simulink model "Simulink_Model"  (R2018a)
settings: Solver=VariableStepAuto  StartTime=0.0  StopTime=T_v(n+1)  MaxStep=0.001
values from neighbouring files (symbols this model uses):
  euler_v = deg2rad(euler_v)    [Simulation_Parameters.m]
  I_b = [151612935.5/10^9	       -12035.62/10^9        -9941.66/10^9 ... (first row only)    [Simulation_Parameters.m]
  I_new = I_sys - I_rw_z * (a1_R1_to_0*a1_0_to_R1+a2_R2_to_0*a2_0_to_R2+a3_R3_to_0*a3_0_to_R3)    [Simulation_Parameters.m]
  I_rw_z = 418129.72/10^9    (= 0.00041812972)    [Simulation_Parameters.m]
  I_single_rw = [220358.07/10^9         0               0 ... (first row only)    [Simulation_Parameters.m]
  I_st = [118601552.74/10^9	       -491524.85/10^9         95420.21/10^9 ... (first row only)    [Simulation_Parameters.m]
  I_sys = [177776253.6/10^9         -12078.47/10^9	        -9914.94/10^9 ... (first row only)    [Simulation_Parameters.m]
  Kd_r = [d;d;d]    [Simulation_Parameters.m]
  Kd_t = [d;d]    [Simulation_Parameters.m]
  Kp_r = [p;p;p]    [Simulation_Parameters.m]
  Kp_t = [p;p]    [Simulation_Parameters.m]
  m_b = 16.9927    [Simulation_Parameters.m]
  m_rw = 0.24806    [Simulation_Parameters.m]
  m_st = 9.48989    [Simulation_Parameters.m]
  m_tot = m_sys + m_st    (= 27.22678)    [Simulation_Parameters.m]
  mf = 1    [Simulation_Parameters.m]
  n = 4    [Simulation_Parameters.m]
  R_0_to_1 = [sqrt(2)/2 0.5 0.5; -sqrt(2)/2 0.5 0.5; 0 -sqrt(2)/2 sqrt(2)/2]    [Simulation_Parameters.m]
  R_1_to_0 = inv(R_0_to_1)    [Simulation_Parameters.m]
undefined symbols (not defined in the file or in its folder): k_phi_1, k_phi_2, k_phi_3, k_psi_1, k_psi_2, k_psi_3, k_theta_1, k_theta_2, k_theta_3, k_x_1, k_x_2, k_x_3, k_y_1, k_y_2, k_y_3, pos_v, t_acc, t_no_acc, t_t_acc, t_t_no_acc, T_v, X, Y, Z
libraries: nesl_utility x20, sm_lib x16, vrlib x2
(part 1 of 2)
settings Model: Creator=menel  LastModifiedBy=Menelaos
settings SolverCC: MaxConsecutiveZCs=10000  ShapePreserveControl=EnableAll  ZeroCrossAlgorithm=Adaptive  AlgebraicLoopSolver=LineSearch
settings DebuggingCC: MaxConsecutiveZCsMsg=none

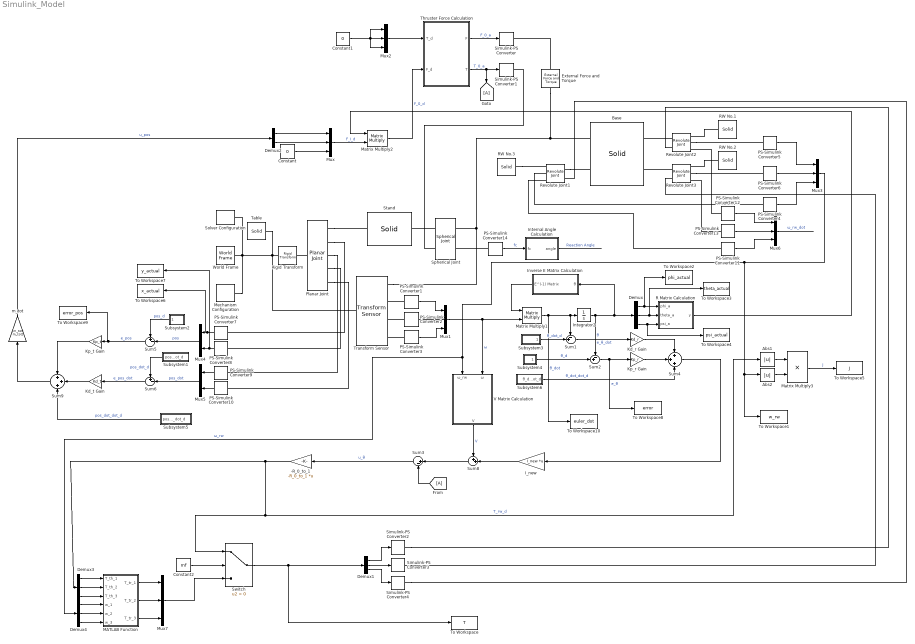
== system Simulink_Model ==
  -R_0_to_1 : Gain  Gain=-R_0_to_1  Multiplication=Matrix(K*u) (u vector)
  Abs1 : Abs
  Abs2 : Abs
  Base : sm_lib/Body Elements/Solid  InertiaType=Custom  Mass=m_b  MassUnits=kg  CenterOfMass=COM_b  CenterOfMassUnits=m  MomentsOfInertia=[I_b(1,1) I_b(2,2) I_b(3,3)]  MomentsOfInertiaUnits=kg*m^2  ProductsOfInertia=[I_b(2,3) I_b(1,3) I_b(2,1)]  ProductsOfInertiaUnits=kg*m^2  DensityBased=off  Density=1000  DensityUnits=kg/m^3  DoExposeReferenceFrame=on  SerializedFrames=<Frames><Frame><Id>Frame1</Id><Value><Name>wheel 1</Name><Origin><Source>GeometricFeature</Source><FeatureName>planar surface 30</FeatureName></Origin><PrimaryAxis><DefinedDirection>+Z</DefinedDirection><Source>GeometricFeature</Source><SourceDirection>+Z</SourceDirection><FeatureName>planar surface 30</FeatureName></PrimaryAxis><SecondaryAxis><DefinedDirection>+X</DefinedDirection><Source>ReferenceFrame</Source><SourceDirection>+X</SourceDirection><FeatureName></FeatureName></SecondaryAxis></Value></Frame><Frame><Id>Frame2</Id><Value><Name>wheel 2</Name><Origin><Source>GeometricFeature</Source><FeatureName>planar surface 29</FeatureName></Origin><PrimaryAxis><DefinedDirection>+Z</DefinedDirection><Source>GeometricFeature</Source><SourceDirection>+Z</SourceDirection><FeatureName>planar surface 29</FeatureName></PrimaryAxis><SecondaryAxis><DefinedDirection>+X</DefinedDirection><Source>ReferenceFrame</Source><SourceDirection>+X</SourceDirection><FeatureName></FeatureName></SecondaryAxis></Value></Frame><Frame><Id>Frame3</Id><Value><Name>wheel 3</Name><Origin><Source>GeometricFeature</Source><FeatureName>planar surface 31</FeatureName></Origin><PrimaryAxis><DefinedDirection>+Z</DefinedDirection><Source>GeometricFeature</Source><SourceDirection>+Z</SourceDirection><FeatureName>planar surface 31</FeatureName></PrimaryAxis><SecondaryAxis><DefinedDirection>+X</DefinedDirection><Source>ReferenceFrame</Source><SourceDirection>+X</SourceDirection><FeatureName></FeatureName></SecondaryAxis></Value></Frame></Frames>  GraphicType=FromGeometry  MarkerShape=Sphere  MarkerSize=10  GraphicVisPropType=SimpleVisualProperties  GraphicDiffuseColor=[0.6 0.6 1.0]  GraphicSpecularColor=[0.5 0.5 0.5 1.0]  GraphicAmbientColor=[0.15 0.15 0.15 1.0]  GraphicEmissiveColor=[0.0 0.0 0.0 1.0]  GraphicShininess=75  GraphicOpacity=1.0  GeometryShape=FromFile  RectangleSize=[1 1]  RectangleSizeUnits=m  BrickDimensions=[1 1 1]  BrickDimensionUnits=m  CylinderRadius=1  CylinderRadiusUnits=m  CylinderLength=1  CylinderLengthUnits=m  SphereRadius=1  SphereRadiusUnits=m  EllipsoidRadii=[1 1 1]  EllipsoidRadiiUnits=m  ExtrusionCrossSection=[1 1; -1 1; -1 -1; 1 -1]  ExtrusionCrossSectionUnits=m  ExtrusionLength=1  ExtrusionLengthUnits=m  PolygonNumSides=3  PolygonOuterRadius=1  PolygonOuterRadiusUnits=m  ExtGeomFileType=STEP  ExtGeomFileName=D:\School\Διπλωματική\Final_Delivery\Motion_and_Rotation_Simulation\Base.STEP  ExtGeomFileUnits=m  RevolutionCrossSection=[1 1; 1 -1; 2 -1; 2 1]  RevolutionCrossSectionUnits=m  RevolutionExtent=Full  RevolutionAngle=180  RevolutionAngleUnits=deg
  Constant : Constant  Value=0
  Constant1 : Constant  Value=0
  Constant2 : Constant  Value=mf
  Demux{,1,3..4} (4 alike) : Demux  Outputs=3
  Demux2 : Demux  Outputs=2
  External Force and Torque : sm_lib/Forces and Torques/External Force and Torque  ForceResolutionFrame=AttachedFrame  EnableForceX=off  EnableForceY=off  EnableForceZ=off  EnableForce=on  TorqueResolutionFrame=AttachedFrame  EnableTorqueX=off  EnableTorqueY=off  EnableTorqueZ=off  EnableTorque=off
  I_new : Gain  Gain=I_new  Multiplication=Matrix(K*u) (u vector)
  Integrator2 : Integrator
  Internal Angle Calculation : MATLAB Function  TreatAsAtomicUnit=on
  Inverse E Matrix Calculation : Subsystem
  Kd_r Gain : Gain  Gain=Kd_r
  Kd_t Gain : Gain  Gain=Kd_t
  Kp_r Gain : Gain  Gain=Kp_r
  Kp_t Gain : Gain  Gain=Kp_t
  MATLAB Function : MATLAB Function  TreatAsAtomicUnit=on
  Matrix Multiply1 : Product  Multiplication=Matrix(*)
  Matrix Multiply2 : Product  Multiplication=Matrix(*)
  Matrix Multiply3 : Product
  Mechanism Configuration : sm_lib/Utilities/Mechanism Configuration  UniformGravity=Constant  GravityVector=[0 0 0]  GravityUnits=m/s^2  LinearizationDelta=0.001
  Mux{,1..3,6..7} (6 alike) : Mux  Inputs=3
  Mux4 : Mux  Inputs=2
  Mux5 : Mux  Inputs=2
  PS-Simulink Converter{1..3,7..13} (10 alike) : nesl_utility/PS-Simulink Converter  PhysicalDomain=network_engine_domain  SubClassName=ps_output  LeftPortType=input  RightPortType=output  PseudoPeriodic=off  Frequencies=[]  Unit=1  AffineConversion=off
  PS-Simulink Converter14 : nesl_utility/PS-Simulink Converter  PhysicalDomain=network_engine_domain  SubClassName=ps_output  LeftPortType=input  RightPortType=output  PseudoPeriodic=off  Frequencies=[]  Unit=N  AffineConversion=off
  PS-Simulink Converter4 : nesl_utility/PS-Simulink Converter  PhysicalDomain=network_engine_domain  SubClassName=ps_output  LeftPortType=input  RightPortType=output  PseudoPeriodic=off  Frequencies=[]  Unit=rad/s  AffineConversion=off
  PS-Simulink Converter5 : nesl_utility/PS-Simulink Converter  PhysicalDomain=network_engine_domain  SubClassName=ps_output  LeftPortType=input  RightPortType=output  PseudoPeriodic=off  Frequencies=[]  Unit=rad/s  AffineConversion=off
  PS-Simulink Converter6 : nesl_utility/PS-Simulink Converter  PhysicalDomain=network_engine_domain  SubClassName=ps_output  LeftPortType=input  RightPortType=output  PseudoPeriodic=off  Frequencies=[]  Unit=rad/s  AffineConversion=off
  Planar Joint : sm_lib/Joints/Planar Joint  SenseConstraintForce=off  SenseConstraintForceX=off  SenseConstraintForceY=off  SenseConstraintForceZ=off  SenseConstraintTorque=off  SenseConstraintTorqueX=off  SenseConstraintTorqueY=off  SenseConstraintTorqueZ=off  SenseTotalForce=off  SenseTotalForceX=off  SenseTotalForceY=off  SenseTotalForceZ=off  SenseTotalTorque=off  SenseTotalTorqueX=off  SenseTotalTorqueY=off  SenseTotalTorqueZ=off  CompositeWrenchDir=FollowerOnBase  CompositeWrenchFrame=BaseFrame  PxEquilibriumPosition=0  PxEquilibriumPositionUnits=m  PxSpringStiffness=0  PxSpringStiffnessUnits=N/m  PxDampingCoefficient=0  PxDampingCoefficientUnits=N/(m/s)  PxTorqueActuationMode=NoTorque  PxMotionActuationMode=ComputedMotion  PxSensePosition=on  PxSenseVelocity=on  PxSenseAcceleration=off  PxSenseTorqueForce=off  PxPositionTargetSpecify=off  PxPositionTargetPriority=High  PxPositionTargetValue=0  PxPositionTargetValueUnits=m  PxVelocityTargetSpecify=off  PxVelocityTargetPriority=High  PxVelocityTargetValue=0  PxVelocityTargetValueUnits=m/s  PyEquilibriumPosition=0  PyEquilibriumPositionUnits=m  PySpringStiffness=0  PySpringStiffnessUnits=N/m  PyDampingCoefficient=0  PyDampingCoefficientUnits=N/(m/s)  PyTorqueActuationMode=NoTorque  PyMotionActuationMode=ComputedMotion  PySensePosition=on  PySenseVelocity=on  PySenseAcceleration=off  PySenseTorqueForce=off  PyPositionTargetSpecify=off  PyPositionTargetPriority=High  PyPositionTargetValue=0  PyPositionTargetValueUnits=m  PyVelocityTargetSpecify=off  PyVelocityTargetPriority=High  PyVelocityTargetValue=0  PyVelocityTargetValueUnits=m/s  RzEquilibriumPosition=0  RzEquilibriumPositionUnits=deg  RzSpringStiffness=100  RzSpringStiffnessUnits=N*m/deg  RzDampingCoefficient=100  RzDampingCoefficientUnits=N*m/(deg/s)  RzTorqueActuationMode=NoTorque  RzMotionActuationMode=ComputedMotion  RzSensePosition=off  RzSenseVelocity=off  RzSenseAcceleration=off  RzSenseTorqueForce=off  RzPositionTargetSpecify=off  RzPositionTargetPriority=High  RzPositionTargetValue=0  RzPositionTargetValueUnits=deg  RzVelocityTargetSpecify=off  RzVelocityTargetPriority=High  RzVelocityTargetValue=0  RzVelocityTargetValueUnits=deg/s
  R Matrix Calculation : MATLAB Function  TreatAsAtomicUnit=on
  RW No.1 : sm_lib/Body Elements/Solid  InertiaType=Custom  Mass=m_rw  MassUnits=kg  CenterOfMass=COM_rw  CenterOfMassUnits=m  MomentsOfInertia=[I_single_rw(1,1) I_single_rw(2,2) I_single_rw(3,3)]  MomentsOfInertiaUnits=kg*m^2  ProductsOfInertia=[I_single_rw(2,3) I_single_rw(1,3) I_single_rw(2,1)]  ProductsOfInertiaUnits=kg*m^2  DensityBased=off  Density=1000  DensityUnits=kg/m^3  DoExposeReferenceFrame=off  SerializedFrames=<Frames><Frame><Id>Frame1</Id><Value><Name>R</Name><Origin><Source>GeometricFeature</Source><FeatureName>planar surface 2</FeatureName></Origin><PrimaryAxis><DefinedDirection>+Z</DefinedDirection><Source>ReferenceFrame</Source><SourceDirection>+Z</SourceDirection><FeatureName></FeatureName></PrimaryAxis><SecondaryAxis><DefinedDirection>+X</DefinedDirection><Source>ReferenceFrame</Source><SourceDirection>+X</SourceDirection><FeatureName></FeatureName></SecondaryAxis></Value></Frame></Frames>  GraphicType=FromGeometry  MarkerShape=Sphere  MarkerSize=10  GraphicVisPropType=SimpleVisualProperties  GraphicDiffuseColor=[1.0 0.2 0.2]  GraphicSpecularColor=[0.5 0.5 0.5 1.0]  GraphicAmbientColor=[0.15 0.15 0.15 1.0]  GraphicEmissiveColor=[0.0 0.0 0.0 1.0]  GraphicShininess=75  GraphicOpacity=1.0  GeometryShape=FromFile  RectangleSize=[1 1]  RectangleSizeUnits=m  BrickDimensions=[1 1 1]  BrickDimensionUnits=m  CylinderRadius=1  CylinderRadiusUnits=m  CylinderLength=1  CylinderLengthUnits=m  SphereRadius=1  SphereRadiusUnits=m  EllipsoidRadii=[1 1 1]  EllipsoidRadiiUnits=m  ExtrusionCrossSection=[1 1; -1 1; -1 -1; 1 -1]  ExtrusionCrossSectionUnits=m  ExtrusionLength=1  ExtrusionLengthUnits=m  PolygonNumSides=3  PolygonOuterRadius=1  PolygonOuterRadiusUnits=m  ExtGeomFileType=STEP  ExtGeomFileName=D:\School\Διπλωματική\Final_Delivery\Motion_and_Rotation_Simulation\Reaction_Wheel.STEP  ExtGeomFileUnits=m  RevolutionCrossSection=[1 1; 1 -1; 2 -1; 2 1]  RevolutionCrossSectionUnits=m  RevolutionExtent=Full  RevolutionAngle=180  RevolutionAngleUnits=deg
  RW No.2 : sm_lib/Body Elements/Solid  InertiaType=Custom  Mass=m_rw  MassUnits=kg  CenterOfMass=COM_rw  CenterOfMassUnits=m  MomentsOfInertia=[I_single_rw(1,1) I_single_rw(2,2) I_single_rw(3,3)]  MomentsOfInertiaUnits=kg*m^2  ProductsOfInertia=[I_single_rw(2,3) I_single_rw(1,3) I_single_rw(2,1)]  ProductsOfInertiaUnits=kg*m^2  DensityBased=off  Density=1000  DensityUnits=kg/m^3  DoExposeReferenceFrame=off  SerializedFrames=<Frames><Frame><Id>Frame1</Id><Value><Name>R</Name><Origin><Source>GeometricFeature</Source><FeatureName>planar surface 2</FeatureName></Origin><PrimaryAxis><DefinedDirection>+Z</DefinedDirection><Source>ReferenceFrame</Source><SourceDirection>+Z</SourceDirection><FeatureName></FeatureName></PrimaryAxis><SecondaryAxis><DefinedDirection>+X</DefinedDirection><Source>ReferenceFrame</Source><SourceDirection>+X</SourceDirection><FeatureName></FeatureName></SecondaryAxis></Value></Frame></Frames>  GraphicType=FromGeometry  MarkerShape=Sphere  MarkerSize=10  GraphicVisPropType=SimpleVisualProperties  GraphicDiffuseColor=[1.0 0.2 0.2]  GraphicSpecularColor=[0.5 0.5 0.5 1.0]  GraphicAmbientColor=[0.15 0.15 0.15 1.0]  GraphicEmissiveColor=[0.0 0.0 0.0 1.0]  GraphicShininess=75  GraphicOpacity=1.0  GeometryShape=FromFile  RectangleSize=[1 1]  RectangleSizeUnits=m  BrickDimensions=[1 1 1]  BrickDimensionUnits=m  CylinderRadius=1  CylinderRadiusUnits=m  CylinderLength=1  CylinderLengthUnits=m  SphereRadius=1  SphereRadiusUnits=m  EllipsoidRadii=[1 1 1]  EllipsoidRadiiUnits=m  ExtrusionCrossSection=[1 1; -1 1; -1 -1; 1 -1]  ExtrusionCrossSectionUnits=m  ExtrusionLength=1  ExtrusionLengthUnits=m  PolygonNumSides=3  PolygonOuterRadius=1  PolygonOuterRadiusUnits=m  ExtGeomFileType=STEP  ExtGeomFileName=D:\School\Διπλωματική\Final_Delivery\Motion_and_Rotation_Simulation\Reaction_Wheel.STEP  ExtGeomFileUnits=m  RevolutionCrossSection=[1 1; 1 -1; 2 -1; 2 1]  RevolutionCrossSectionUnits=m  RevolutionExtent=Full  RevolutionAngle=180  RevolutionAngleUnits=deg
  RW No.3 : sm_lib/Body Elements/Solid  InertiaType=Custom  Mass=m_rw  MassUnits=kg  CenterOfMass=COM_rw  CenterOfMassUnits=m  MomentsOfInertia=[I_single_rw(1,1) I_single_rw(2,2) I_single_rw(3,3)]  MomentsOfInertiaUnits=kg*m^2  ProductsOfInertia=[I_single_rw(2,3) I_single_rw(1,3) I_single_rw(2,1)]  ProductsOfInertiaUnits=kg*m^2  DensityBased=off  Density=1000  DensityUnits=kg/m^3  DoExposeReferenceFrame=off  SerializedFrames=<Frames><Frame><Id>Frame1</Id><Value><Name>R</Name><Origin><Source>GeometricFeature</Source><FeatureName>planar surface 2</FeatureName></Origin><PrimaryAxis><DefinedDirection>+Z</DefinedDirection><Source>ReferenceFrame</Source><SourceDirection>+Z</SourceDirection><FeatureName></FeatureName></PrimaryAxis><SecondaryAxis><DefinedDirection>+X</DefinedDirection><Source>ReferenceFrame</Source><SourceDirection>+X</SourceDirection><FeatureName></FeatureName></SecondaryAxis></Value></Frame></Frames>  GraphicType=FromGeometry  MarkerShape=Sphere  MarkerSize=10  GraphicVisPropType=SimpleVisualProperties  GraphicDiffuseColor=[1.0 0.2 0.2]  GraphicSpecularColor=[0.5 0.5 0.5 1.0]  GraphicAmbientColor=[0.15 0.15 0.15 1.0]  GraphicEmissiveColor=[0.0 0.0 0.0 1.0]  GraphicShininess=75  GraphicOpacity=1.0  GeometryShape=FromFile  RectangleSize=[1 1]  RectangleSizeUnits=m  BrickDimensions=[1 1 1]  BrickDimensionUnits=m  CylinderRadius=1  CylinderRadiusUnits=m  CylinderLength=1  CylinderLengthUnits=m  SphereRadius=1  SphereRadiusUnits=m  EllipsoidRadii=[1 1 1]  EllipsoidRadiiUnits=m  ExtrusionCrossSection=[1 1; -1 1; -1 -1; 1 -1]  ExtrusionCrossSectionUnits=m  ExtrusionLength=1  ExtrusionLengthUnits=m  PolygonNumSides=3  PolygonOuterRadius=1  PolygonOuterRadiusUnits=m  ExtGeomFileType=STEP  ExtGeomFileName=D:\School\Διπλωματική\Final_Delivery\Motion_and_Rotation_Simulation\Reaction_Wheel.STEP  ExtGeomFileUnits=m  RevolutionCrossSection=[1 1; 1 -1; 2 -1; 2 1]  RevolutionCrossSectionUnits=m  RevolutionExtent=Full  RevolutionAngle=180  RevolutionAngleUnits=deg
  Revolute Joint1 : sm_lib/Joints/Revolute Joint  SenseConstraintForce=off  SenseConstraintForceX=off  SenseConstraintForceY=off  SenseConstraintForceZ=off  SenseConstraintTorque=off  SenseConstraintTorqueX=off  SenseConstraintTorqueY=off  SenseConstraintTorqueZ=off  SenseTotalForce=off  SenseTotalForceX=off  SenseTotalForceY=off  SenseTotalForceZ=off  SenseTotalTorque=off  SenseTotalTorqueX=off  SenseTotalTorqueY=off  SenseTotalTorqueZ=off  CompositeWrenchDir=FollowerOnBase  CompositeWrenchFrame=BaseFrame  EquilibriumPosition=0  EquilibriumPositionUnits=deg  SpringStiffness=0  SpringStiffnessUnits=N*m/deg  DampingCoefficient=1.86*10^(-5)  DampingCoefficientUnits=N*m/(rad/s)  TorqueActuationMode=InputTorque  MotionActuationMode=ComputedMotion  SensePosition=off  SenseVelocity=on  SenseAcceleration=on  SenseTorqueForce=off  PositionTargetSpecify=on  PositionTargetPriority=High  PositionTargetValue=0  PositionTargetValueUnits=deg  VelocityTargetSpecify=off  VelocityTargetPriority=High  VelocityTargetValue=300  VelocityTargetValueUnits=rad/s
  Revolute Joint2 : sm_lib/Joints/Revolute Joint  SenseConstraintForce=off  SenseConstraintForceX=off  SenseConstraintForceY=off  SenseConstraintForceZ=off  SenseConstraintTorque=off  SenseConstraintTorqueX=off  SenseConstraintTorqueY=off  SenseConstraintTorqueZ=off  SenseTotalForce=off  SenseTotalForceX=off  SenseTotalForceY=off  SenseTotalForceZ=off  SenseTotalTorque=off  SenseTotalTorqueX=off  SenseTotalTorqueY=off  SenseTotalTorqueZ=off  CompositeWrenchDir=FollowerOnBase  CompositeWrenchFrame=BaseFrame  EquilibriumPosition=0  EquilibriumPositionUnits=deg  SpringStiffness=0  SpringStiffnessUnits=N*m/deg  DampingCoefficient=1.86*10^(-5)  DampingCoefficientUnits=N*m/(rad/s)  TorqueActuationMode=InputTorque  MotionActuationMode=ComputedMotion  SensePosition=off  SenseVelocity=on  SenseAcceleration=on  SenseTorqueForce=off  PositionTargetSpecify=on  PositionTargetPriority=High  PositionTargetValue=0  PositionTargetValueUnits=deg  VelocityTargetSpecify=off  VelocityTargetPriority=High  VelocityTargetValue=300  VelocityTargetValueUnits=rad/s
  Revolute Joint3 : sm_lib/Joints/Revolute Joint  SenseConstraintForce=off  SenseConstraintForceX=off  SenseConstraintForceY=off  SenseConstraintForceZ=off  SenseConstraintTorque=off  SenseConstraintTorqueX=off  SenseConstraintTorqueY=off  SenseConstraintTorqueZ=off  SenseTotalForce=off  SenseTotalForceX=off  SenseTotalForceY=off  SenseTotalForceZ=off  SenseTotalTorque=off  SenseTotalTorqueX=off  SenseTotalTorqueY=off  SenseTotalTorqueZ=off  CompositeWrenchDir=FollowerOnBase  CompositeWrenchFrame=BaseFrame  EquilibriumPosition=0  EquilibriumPositionUnits=deg  SpringStiffness=0  SpringStiffnessUnits=N*m/deg  DampingCoefficient=1.86*10^(-5)  DampingCoefficientUnits=N*m/(rad/s)  TorqueActuationMode=InputTorque  MotionActuationMode=ComputedMotion  SensePosition=off  SenseVelocity=on  SenseAcceleration=on  SenseTorqueForce=off  PositionTargetSpecify=on  PositionTargetPriority=High  PositionTargetValue=0  PositionTargetValueUnits=deg  VelocityTargetSpecify=off  VelocityTargetPriority=High  VelocityTargetValue=300  VelocityTargetValueUnits=rad/s
  Rigid Transform : sm_lib/Frames and Transforms/Rigid Transform  TranslationMethod=StandardAxis  TranslationStandardOffset=46  TranslationLengthUnit=mm  TranslationStandardAxis=+Z  TranslationCartesianOffset=[0 0 0]  TranslationROffset=0  TranslationROffsetUnits=m  TranslationZOffset=0  TranslationZOffsetUnits=m  TranslationThetaOffset=0  TranslationThetaOffsetUnits=deg  RotationMethod=None  RotationAngleUnits=deg  RotationStandardAxis=+Z  RotationAngle=0.0  RotationArbitraryAxis=[0 0 1]  FollAlignAxisA=+X  BaseAlignAxisA=+Y  FollAlignAxisB=+Y  BaseAlignAxisB=+Z  RotationSequenceAxes=FollowerAxes  RotationSequence=XYX  RotationSequenceAngles=[0 0 0]  RotationSequenceAnglesUnits=deg  RotationMatrix=[1 0 0; 0 1 0; 0 0 1]
  Simulink-PS Converter : nesl_utility/Simulink-PS Converter  PhysicalDomain=network_engine_domain  SubClassName=ps_input  LeftPortType=input  RightPortType=output  PseudoPeriodic=off  Frequencies=[]  NoiseDistribution=none  NoiseParameters=[]  Unit=1  AffineConversion=off  FilteringAndDerivatives=provide  SimscapeFilterOrder=1  InputFilterTimeConstant=0.001  UdotUserProvided=0
  Simulink-PS Converter1 : nesl_utility/Simulink-PS Converter  PhysicalDomain=network_engine_domain  SubClassName=ps_input  LeftPortType=input  RightPortType=output  PseudoPeriodic=off  Frequencies=[]  NoiseDistribution=none  NoiseParameters=[]  Unit=1  AffineConversion=off  FilteringAndDerivatives=provide  SimscapeFilterOrder=1  InputFilterTimeConstant=0.001  UdotUserProvided=0
  Simulink-PS Converter2 : nesl_utility/Simulink-PS Converter  PhysicalDomain=network_engine_domain  SubClassName=ps_input  LeftPortType=input  RightPortType=output  PseudoPeriodic=off  Frequencies=[]  NoiseDistribution=none  NoiseParameters=[]  Unit=N*m  AffineConversion=off  FilteringAndDerivatives=zero  SimscapeFilterOrder=1  InputFilterTimeConstant=0.001  UdotUserProvided=1
  Simulink-PS Converter3 : nesl_utility/Simulink-PS Converter  PhysicalDomain=network_engine_domain  SubClassName=ps_input  LeftPortType=input  RightPortType=output  PseudoPeriodic=off  Frequencies=[]  NoiseDistribution=none  NoiseParameters=[]  Unit=N*m  AffineConversion=off  FilteringAndDerivatives=zero  SimscapeFilterOrder=1  InputFilterTimeConstant=0.001  UdotUserProvided=1
  Simulink-PS Converter4 : nesl_utility/Simulink-PS Converter  PhysicalDomain=network_engine_domain  SubClassName=ps_input  LeftPortType=input  RightPortType=output  PseudoPeriodic=off  Frequencies=[]  NoiseDistribution=none  NoiseParameters=[]  Unit=N*m  AffineConversion=off  FilteringAndDerivatives=zero  SimscapeFilterOrder=1  InputFilterTimeConstant=0.001  UdotUserProvided=1
  Solver Configuration : nesl_utility/Solver Configuration  PhysicalDomain=network_engine_domain  SubClassName=solver  LeftPortType=input  RightPortType=generic  Tones=[]  Harmonics=[]  SimulateNoise=off  Profile=off  UseLocalSampling=off  EnableSwitchedLinearOptims=on  FrequencyDomain=off  UseCCode=off  RelTol=0.001  AbsTol=1e-06  MinStep=1e-09  ToWorkspace=off  RevertToSquareIcSolve=off  NumHomotopyIterations=100  PhasorMode=off  PhasorModeNumHarmonics=1  DoDC=off  ResidualTolerance=1e-09  UseLocalSolver=off  LocalSolverChoice=NE_BACKWARD_EULER_ADVANCER  LocalSolverSampleTime=0.001  DoFixedCost=off  MaxNonlinIter=3  MaxModeIter=2  LinearAlgebra=Sparse  EquationFormulation=NE_TIME_EF  DelaysMemoryBudget=1024  AutomaticFiltering=on  FilteringTimeConstant=0.001
  Spherical Joint : sm_lib/Joints/Spherical Joint  SenseConstraintForce=on  SenseConstraintForceX=off  SenseConstraintForceY=off  SenseConstraintForceZ=off  SenseConstraintTorque=off  SenseConstraintTorqueX=off  SenseConstraintTorqueY=off  SenseConstraintTorqueZ=off  SenseTotalForce=off  SenseTotalForceX=off  SenseTotalForceY=off  SenseTotalForceZ=off  SenseTotalTorque=off  SenseTotalTorqueX=off  SenseTotalTorqueY=off  SenseTotalTorqueZ=off  CompositeWrenchDir=FollowerOnBase  CompositeWrenchFrame=BaseFrame  DefPosRotationMethod=None  DefPosRotationAngleUnits=deg  DefPosRotationStandardAxis=+Z  DefPosRotationAngle=0.0  DefPosRotationArbitraryAxis=[0 0 1]  DefPosFollAlignAxisA=+X  DefPosBaseAlignAxisA=+Y  DefPosFollAlignAxisB=+Y  DefPosBaseAlignAxisB=+Z  DefPosRotationSequenceAxes=FollowerAxes  DefPosRotationSequence=XYX  DefPosRotationSequenceAngles=[0 0 0]  DefPosRotationSequenceAnglesUnits=deg  DefPosRotationMatrix=[1 0 0; 0 1 0; 0 0 1]  EqPosRotationMethod=None  EqPosRotationAngleUnits=deg  EqPosRotationStandardAxis=+Z  EqPosRotationAngle=0.0  EqPosRotationArbitraryAxis=[0 0 1]  EqPosFollAlignAxisA=+X  EqPosBaseAlignAxisA=+Y  EqPosFollAlignAxisB=+Y  EqPosBaseAlignAxisB=+Z  EqPosRotationSequenceAxes=FollowerAxes  EqPosRotationSequence=XYX  EqPosRotationSequenceAngles=[0 0 0]  EqPosRotationSequenceAnglesUnits=deg  EqPosRotationMatrix=[1 0 0; 0 1 0; 0 0 1]  SpringStiffness=0  SpringStiffnessUnits=N*m/deg  DampingCoefficient=0  DampingCoefficientUnits=N*m/(deg/s)  ActuateTorqueX=off  ActuateTorqueY=off  ActuateTorqueZ=off  ActuateTorque=on  TorqueActuationMode=InputTorque  MotionActuationMode=ComputedMotion  ActuationFrame=FollowerFrame  SensePosition=off  SenseVelocityX=off  SenseVelocityY=off  SenseVelocityZ=off  SenseVelocity=off  SenseAccelerationX=off  SenseAccelerationY=off  SenseAccelerationZ=off  SenseAcceleration=off  SenseTorqueX=off  SenseTorqueY=off  SenseTorqueZ=off  SenseTorqueForce=off  SensingFrame=FollowerFrame  PositionTargetRotationMethod=None  PositionTargetRotationAngleUnits=deg  PositionTargetRotationStandardAxis=+Z  PositionTargetRotationAngle=0.0  PositionTargetRotationArbitraryAxis=[0 0 1]  PositionTargetFollAlignAxisA=+X  PositionTargetBaseAlignAxisA=+Y  PositionTargetFollAlignAxisB=+Y  PositionTargetBaseAlignAxisB=+Z  PositionTargetRotationSequenceAxes=FollowerAxes  PositionTargetRotationSequence=XYX  PositionTargetRotationSequenceAngles=[0 0 0]  PositionTargetRotationSequenceAnglesUnits=deg  PositionTargetRotationMatrix=[1 0 0; 0 1 0; 0 0 1]  PositionTargetSpecify=off  PositionTargetPriority=High  VelocityTargetValue=[0 0 0]  VelocityTargetValueUnits=deg/s  VelocityTargetSpecify=off  VelocityTargetPriority=High  VelocityTargetInFollowerFrame=on
  Stand : sm_lib/Body Elements/Solid  InertiaType=Custom  Mass=m_st  MassUnits=kg  CenterOfMass=COM_st  CenterOfMassUnits=m  MomentsOfInertia=[I_st(1,1) I_st(2,2) I_st(3,3)]  MomentsOfInertiaUnits=kg*m^2  ProductsOfInertia=[I_st(2,3) I_st(1,3) I_st(2,1)]  ProductsOfInertiaUnits=kg*m^2  DensityBased=on  Density=1000  DensityUnits=kg/m^3  DoExposeReferenceFrame=on  SerializedFrames=<Frames><Frame><Id>Frame1</Id><Value><Name>Rotation Frame</Name><Origin><Source>GeometricFeature</Source><FeatureName>spherical surface 1</FeatureName></Origin><PrimaryAxis><DefinedDirection>+Z</DefinedDirection><Source>ReferenceFrame</Source><SourceDirection>+Z</SourceDirection><FeatureName></FeatureName></PrimaryAxis><SecondaryAxis><DefinedDirection>+X</DefinedDirection><Source>ReferenceFrame</Source><SourceDirection>+X</SourceDirection><FeatureName></FeatureName></SecondaryAxis></Value></Frame></Frames>  GraphicType=FromGeometry  MarkerShape=Sphere  MarkerSize=10  GraphicVisPropType=SimpleVisualProperties  GraphicDiffuseColor=[1.0 0.2 0.2]  GraphicSpecularColor=[0.5 0.5 0.5 1.0]  GraphicAmbientColor=[0.15 0.15 0.15 1.0]  GraphicEmissiveColor=[0.0 0.0 0.0 1.0]  GraphicShininess=75  GraphicOpacity=1.0  GeometryShape=FromFile  RectangleSize=[1 1]  RectangleSizeUnits=m  BrickDimensions=[1 1 1]  BrickDimensionUnits=m  CylinderRadius=1  CylinderRadiusUnits=m  CylinderLength=1  CylinderLengthUnits=m  SphereRadius=1  SphereRadiusUnits=m  EllipsoidRadii=[1 1 1]  EllipsoidRadiiUnits=m  ExtrusionCrossSection=[1 1; -1 1; -1 -1; 1 -1]  ExtrusionCrossSectionUnits=m  ExtrusionLength=1  ExtrusionLengthUnits=m  PolygonNumSides=3  PolygonOuterRadius=1  PolygonOuterRadiusUnits=m  ExtGeomFileType=STEP  ExtGeomFileName=D:\School\Διπλωματική\Final_Delivery\Motion_and_Rotation_Simulation\Stand.STEP  ExtGeomFileUnits=m  RevolutionCrossSection=[1 1; 1 -1; 2 -1; 2 1]  RevolutionCrossSectionUnits=m  RevolutionExtent=Full  RevolutionAngle=180  RevolutionAngleUnits=deg
  Subsystem1 : Subsystem
  Subsystem2 : Subsystem
  Subsystem3 : Subsystem
  Subsystem4 : Subsystem
  Subsystem5 : Subsystem
  Subsystem6 : Subsystem
  Sum1 : Sum  Inputs=-+|
  Sum2 : Sum  Inputs=-+|
  Sum3 : Sum  Inputs=|+-
  Sum4 : Sum  Inputs=+++
  Sum5 : Sum  Inputs=+-|
  Sum6 : Sum  Inputs=+-|
  Sum8 : Sum  Inputs=++|
  Sum9 : Sum  Inputs=+++
  Switch : Switch  Criteria=u2 > Threshold
  Table : sm_lib/Body Elements/Solid  InertiaType=CalculateFromGeometry  Mass=1  MassUnits=kg  CenterOfMass=[0 0 0]  CenterOfMassUnits=m  MomentsOfInertia=[1 1 1]  MomentsOfInertiaUnits=kg*m^2  ProductsOfInertia=[0 0 0]  ProductsOfInertiaUnits=kg*m^2  DensityBased=on  Density=1000  DensityUnits=kg/m^3  DoExposeReferenceFrame=on  SerializedFrames=<Frames/>  GraphicType=FromGeometry  MarkerShape=Sphere  MarkerSize=10  GraphicVisPropType=SimpleVisualProperties  GraphicDiffuseColor=[0.5 0.5 0.5]  GraphicSpecularColor=[0.5 0.5 0.5 1.0]  GraphicAmbientColor=[0.15 0.15 0.15 1.0]  GraphicEmissiveColor=[0.0 0.0 0.0 1.0]  GraphicShininess=75  GraphicOpacity=1.0  GeometryShape=FromFile  RectangleSize=[1 1]  RectangleSizeUnits=m  BrickDimensions=[1 1 1]  BrickDimensionUnits=m  CylinderRadius=1  CylinderRadiusUnits=m  CylinderLength=1  CylinderLengthUnits=m  SphereRadius=1  SphereRadiusUnits=m  EllipsoidRadii=[1 1 1]  EllipsoidRadiiUnits=m  ExtrusionCrossSection=[1 1; -1 1; -1 -1; 1 -1]  ExtrusionCrossSectionUnits=m  ExtrusionLength=1  ExtrusionLengthUnits=m  PolygonNumSides=3  PolygonOuterRadius=1  PolygonOuterRadiusUnits=m  ExtGeomFileType=STEP  ExtGeomFileName=D:\School\Διπλωματική\Final_Delivery\Motion_and_Rotation_Simulation\Table.STEP  ExtGeomFileUnits=m  RevolutionCrossSection=[1 1; 1 -1; 2 -1; 2 1]  RevolutionCrossSectionUnits=m  RevolutionExtent=Full  RevolutionAngle=180  RevolutionAngleUnits=deg
  Thruster Force Calculation : Subsystem
  To Workspace : ToWorkspace  VariableName=T  SampleTime=-1
  To Workspace1 : ToWorkspace  VariableName=w_rw  SampleTime=-1
  To Workspace10 : ToWorkspace  VariableName=euler_dot  SampleTime=-1
  To Workspace2 : ToWorkspace  VariableName=phi_actual  SaveFormat=Timeseries  SampleTime=-1
      settings: Save2DSignal=2-D array (concatenate along first dimension)
  To Workspace3 : ToWorkspace  VariableName=theta_actual  SaveFormat=Timeseries  SampleTime=-1
      settings: Save2DSignal=2-D array (concatenate along first dimension)
  To Workspace4 : ToWorkspace  VariableName=psi_actual  SaveFormat=Timeseries  SampleTime=-1
      settings: Save2DSignal=2-D array (concatenate along first dimension)
  To Workspace5 : ToWorkspace  VariableName=J  SampleTime=-1
  To Workspace6 : ToWorkspace  VariableName=x_actual  SaveFormat=Timeseries  SampleTime=-1
      settings: Save2DSignal=2-D array (concatenate along first dimension)
  To Workspace7 : ToWorkspace  VariableName=y_actual  SaveFormat=Timeseries  SampleTime=-1
      settings: Save2DSignal=2-D array (concatenate along first dimension)
  To Workspace8 : ToWorkspace  VariableName=error  SampleTime=-1
  To Workspace9 : ToWorkspace  VariableName=error_pos  SampleTime=-1
  Transform Sensor : sm_lib/Frames and Transforms/Transform Sensor  MeasurementFrame=Follower  SenseAngle=off  SenseAxis=off  SenseAngle1=off  SenseAngle2=off  SenseAngle3=off  SenseQ=off  SenseR=off  SenseOmegaX=on  SenseOmegaY=on  SenseOmegaZ=on  SenseOmega1=off  SenseOmega2=off  SenseOmega3=off  SenseQDot=off  SenseRDot=off  SenseAlphaX=off  SenseAlphaY=off  SenseAlphaZ=off  SenseAlpha1=off  SenseAlpha2=off  SenseAlpha3=off  SenseQDDot=off  SenseRDDot=off  SenseX=off  SenseY=off  SenseZ=off  SenseRad=off  SenseAzim=off  SenseDist=off  SenseInc=off  SenseXDot=off  SenseYDot=off  SenseZDot=off  SenseRadDot=off  SenseAzimDot=off  SenseDistDot=off  SenseIncDot=off  SenseXDDot=off  SenseYDDot=off  SenseZDDot=off  SenseRadDDot=off  SenseAzimDDot=off  SenseDistDDot=off  SenseIncDDot=off
  V Matrix Calculation : Subsystem
  World Frame : sm_lib/Frames and Transforms/World Frame
  m_tot : Gain  Gain=[m_tot; m_tot]
  wires:
  Inverse E Matrix Calculation/1(E^(-1) Matrix) -> Matrix Multiply1/1
  Matrix Multiply1/1 -> To Workspace10/1, Sum1/1, Integrator2/1  "θ_dot"
  Integrator2/1 -> Demux/1, Inverse E Matrix Calculation/1(θ), Sum2/1  "θ"
  Demux/2 -> To Workspace3/1, R Matrix Calculation/2(theta_a)
  Demux/1 -> To Workspace2/1, R Matrix Calculation/1(phi_a)
  Demux/3 -> To Workspace4/1, R Matrix Calculation/3(psi_a)
  Mux/1 -> Matrix Multiply2/2  "F_I_d"
  R Matrix Calculation/1(y) -> Matrix Multiply2/1
  Mux1/1 -> Matrix Multiply1/2, V Matrix Calculation/2(ω)  "ω"
  PS-Simulink Converter2/1 -> Mux1/2
  PS-Simulink Converter1/1 -> Mux1/1
  PS-Simulink Converter3/1 -> Mux1/3
  Constant1/1 -> Mux2/3, Mux2/1, Mux2/2
  Matrix Multiply2/1 -> Thruster Force Calculation/2(F_d)  "F_0_d"
  Thruster Force Calculation/1(F) -> Simulink-PS Converter/1  "F_0_a"
  Thruster Force Calculation/2(T) -> [A], Simulink-PS Converter1/1  "T_0_a"
  Subsystem3/1(θ_dot_d) -> Sum1/2  "θ_dot_d"
  Subsystem4/1(θ_d) -> Sum2/2  "θ_d"
  Sum2/1 -> To Workspace8/1, Kp_r Gain/1  "e_θ"
  Subsystem6/1(θ_dot_dot_d) -> Sum4/3  "θ_dot_dot_d"
  Sum1/1 -> Kd_r Gain/1  "e_θ_dot"
  Sum4/1 -> I_new/1
  I_new/1 -> Sum8/2
  V Matrix Calculation/1(V) -> Sum8/1  "V"
  PS-Simulink Converter6/1 -> Mux3/2
  PS-Simulink Converter5/1 -> Mux3/1
  PS-Simulink Converter4/1 -> Mux3/3
  Mux3/1 -> To Workspace1/1, Abs2/1, Demux4/1, V Matrix Calculation/1(ω_rw)  "ω_rw"
  [A] -> Sum3/2
  Demux1/2 -> Simulink-PS Converter3/1
  Demux1/3 -> Simulink-PS Converter4/1
  Demux1/1 -> Simulink-PS Converter2/1
  Mux2/1 -> Thruster Force Calculation/1(T_d)
  PS-Simulink Converter7/1 -> To Workspace6/1, Mux4/1
  PS-Simulink Converter8/1 -> To Workspace7/1, Mux4/2
  PS-Simulink Converter9/1 -> Mux5/1
  PS-Simulink Converter10/1 -> Mux5/2
  Mux4/1 -> Sum5/2  "pos"
  Subsystem2/1(pos_d) -> Sum5/1  "pos_d"
  Mux5/1 -> Sum6/2  "pos_dot"
  Subsystem1/1(pos_dot_d) -> Sum6/1  "pos_dot_d"
  Subsystem5/1(pos_dot_dot_d) -> Sum9/3  "pos_dot_dot_d"
  Kp_r Gain/1 -> Sum4/2
  Kd_r Gain/1 -> Sum4/1
  Sum5/1 -> To Workspace9/1, Kp_t Gain/1  "e_pos"
  Kp_t Gain/1 -> Sum9/1
  Kd_t Gain/1 -> Sum9/2
  Sum6/1 -> Kd_t Gain/1  "e_pos_dot"
  Constant/1 -> Mux/3
  Sum9/1 -> m_tot/1
  Sum8/1 -> Sum3/1
  Sum3/1 -> -R_0_to_1/1  "u_θ"
  PS-Simulink Converter12/1 -> Mux6/1
  PS-Simulink Converter13/1 -> Mux6/2
  PS-Simulink Converter11/1 -> Mux6/3
  Mux6/1 -> ?  "ω_rw_dot"
  PS-Simulink Converter14/1 -> Internal Angle Calculation/1(fc)  "fc"
  Internal Angle Calculation/1(angle) -> ?  "Reaction Angle"
  Abs1/1 -> Matrix Multiply3/1
  Matrix Multiply3/1 -> To Workspace5/1  "J"
  Abs2/1 -> Matrix Multiply3/2
  -R_0_to_1/1 -> Demux3/1, Switch/1, Abs1/1  "T_rw_d"
  m_tot/1 -> Demux2/1  "u_pos"
  Demux2/2 -> Mux/2
  Demux2/1 -> Mux/1
  Demux3/1 -> MATLAB Function/1(T_th_1)
  Demux3/2 -> MATLAB Function/2(T_th_2)
  Demux3/3 -> MATLAB Function/3(T_th_3)
  Demux4/1 -> MATLAB Function/4(w_1)
  Demux4/2 -> MATLAB Function/5(w_2)
  Demux4/3 -> MATLAB Function/6(w_3)
  MATLAB Function/2(T_tr_2) -> Mux7/2
  MATLAB Function/1(T_tr_1) -> Mux7/1
  MATLAB Function/3(T_tr_3) -> Mux7/3
  Constant2/1 -> Switch/2
  Switch/1 -> To Workspace/1, Demux1/1
  Mux7/1 -> Switch/3
  connections:
  World Frame/RConn1 -- Mechanism Configuration/RConn1 -- Transform Sensor/LConn1 -- Table/RConn1 -- Rigid Transform/LConn1 -- Solver Configuration/RConn1
  Planar Joint/RConn1 -- Stand/RConn1
  Planar Joint/LConn1 -- Rigid Transform/RConn1
  Spherical Joint/LConn1 -- Stand/LConn1
  External Force and Torque/LConn1 -- Simulink-PS Converter/RConn1
  PS-Simulink Converter2/LConn1 -- Transform Sensor/RConn3
  PS-Simulink Converter1/LConn1 -- Transform Sensor/RConn2
  PS-Simulink Converter3/LConn1 -- Transform Sensor/RConn4
  Revolute Joint1/LConn1 -- Base/RConn2
  RW No.3/LConn1 -- Revolute Joint1/RConn1
  Revolute Joint2/LConn1 -- Base/LConn1
  Revolute Joint3/LConn1 -- Base/LConn2
  RW No.1/LConn1 -- Revolute Joint2/RConn1
  RW No.2/LConn1 -- Revolute Joint3/RConn1
  Spherical Joint/LConn2 -- Simulink-PS Converter1/RConn1
  Revolute Joint2/RConn2 -- PS-Simulink Converter5/LConn1
  Revolute Joint3/RConn2 -- PS-Simulink Converter6/LConn1
  PS-Simulink Converter4/LConn1 -- Revolute Joint1/RConn2
  Simulink-PS Converter2/RConn1 -- Revolute Joint2/LConn2
  Simulink-PS Converter3/RConn1 -- Revolute Joint3/LConn2
  Simulink-PS Converter4/RConn1 -- Revolute Joint1/LConn2
  Planar Joint/RConn2 -- PS-Simulink Converter7/LConn1
  Planar Joint/RConn4 -- PS-Simulink Converter8/LConn1
  Planar Joint/RConn3 -- PS-Simulink Converter9/LConn1
  Planar Joint/RConn5 -- PS-Simulink Converter10/LConn1
  PS-Simulink Converter12/LConn1 -- Revolute Joint2/RConn3
  PS-Simulink Converter13/LConn1 -- Revolute Joint3/RConn3
  PS-Simulink Converter11/LConn1 -- Revolute Joint1/RConn3
  PS-Simulink Converter14/LConn1 -- Spherical Joint/RConn2
  Spherical Joint/RConn1 -- Transform Sensor/RConn1 -- External Force and Torque/RConn1 -- Base/RConn1

== system Simulink_Model/Inverse E Matrix Calculation ==
  θ : Inport
  Demux : Demux  Outputs=3
  E^(-1) Matrix Calculation : MATLAB Function  TreatAsAtomicUnit=on
  E^(-1) Matrix : Outport
  wires:
  Demux/2 -> E^(-1) Matrix Calculation/2(theta_a)  "theta"
  Demux/1 -> E^(-1) Matrix Calculation/1(phi_a)  "phi"
  Demux/3 -> E^(-1) Matrix Calculation/3(psi_a)  "psi"
  θ/1 -> Demux/1
  E^(-1) Matrix Calculation/1(y) -> E^(-1) Matrix/1

== system Simulink_Model/Subsystem1 ==
  Desired x velocity calculation : Subsystem
  Desired y velocity calculation : Subsystem
  Mux : Mux  Inputs=2
  pos_dot_d : Outport
  wires:
  Desired y velocity calculation/1(Out1) -> Mux/2
  Mux/1 -> pos_dot_d/1
  Desired x velocity calculation/1(Out1) -> Mux/1

== system Simulink_Model/Subsystem2 ==
  Desired x position calculation : Subsystem
  Desired y position calculation : Subsystem
  Mux : Mux  Inputs=2
  pos_d : Outport
  wires:
  Mux/1 -> pos_d/1
  Desired y position calculation/1(Out1) -> Mux/2
  Desired x position calculation/1(Out1) -> Mux/1

== system Simulink_Model/Subsystem3 ==
  Desired phi angular velocity calculation : Subsystem
  Desired psi angular velocity calculation : Subsystem
  Desired theta angular velocity calculation : Subsystem
  Mux : Mux  Inputs=3
  θ_dot_d : Outport
  wires:
  Desired theta angular velocity calculation/1(Out1) -> Mux/2
  Desired psi angular velocity calculation/1(Out1) -> Mux/3
  Desired phi angular velocity calculation/1(Out1) -> Mux/1
  Mux/1 -> θ_dot_d/1

== system Simulink_Model/Subsystem4 ==
  Desired phi angle calculation : Subsystem
  Desired psi angle calculation : Subsystem
  Desired theta angle calculation : Subsystem
  Mux : Mux  Inputs=3
  θ_d : Outport
  wires:
  Desired theta angle calculation/1(Out1) -> Mux/2
  Mux/1 -> θ_d/1
  Desired psi angle calculation/1(Out1) -> Mux/3
  Desired phi angle calculation/1(Out1) -> Mux/1

== system Simulink_Model/Subsystem5 ==
  Desired x acceleration calculation : Subsystem
  Desired y acceleration calculation : Subsystem
  Mux : Mux  Inputs=2
  pos_dot_dot_d : Outport
  wires:
  Desired y acceleration calculation/1(Out1) -> Mux/2
  Mux/1 -> pos_dot_dot_d/1
  Desired x acceleration calculation/1(Out1) -> Mux/1

== system Simulink_Model/Subsystem6 ==
  Desired phi angular acceleration calculation : Subsystem
  Desired psi angular acceleration calculation : Subsystem
  Desired theta angular acceleration calculation : Subsystem
  Mux : Mux  Inputs=3
  θ_dot_dot_d : Outport
  wires:
  Desired theta angular acceleration calculation/1(Out1) -> Mux/2
  Desired psi angular acceleration calculation/1(Out1) -> Mux/3
  Desired phi angular acceleration calculation/1(Out1) -> Mux/1
  Mux/1 -> θ_dot_dot_d/1

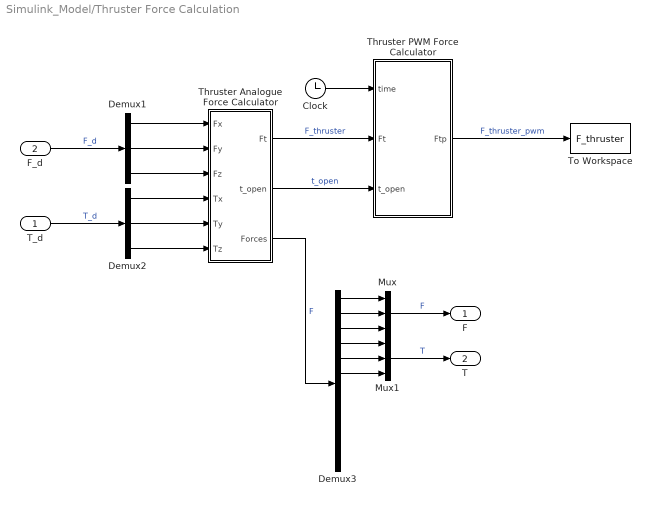
== system Simulink_Model/Thruster Force Calculation ==
  T_d : Inport
  F_d : Inport  Port=2
  Clock : Clock
  Demux1 : Demux  Outputs=3
  Demux2 : Demux  Outputs=3
  Demux3 : Demux  Outputs=12
  Mux : Mux  Inputs=3
  Mux1 : Mux  Inputs=3
  Thruster Analogue Force Calculator : MATLAB Function  TreatAsAtomicUnit=on
  Thruster PWM Force Calculator : MATLAB Function  TreatAsAtomicUnit=on
  To Workspace : ToWorkspace  VariableName=F_thruster  SampleTime=-1
      settings: Save2DSignal=2-D array (concatenate along first dimension)
  F : Outport
  T : Outport  Port=2
  wires:
  Demux2/3 -> Thruster Analogue Force Calculator/6(Tz)
  Demux1/3 -> Thruster Analogue Force Calculator/3(Fz)
  Demux2/1 -> Thruster Analogue Force Calculator/4(Tx)
  Demux1/2 -> Thruster Analogue Force Calculator/2(Fy)
  Demux1/1 -> Thruster Analogue Force Calculator/1(Fx)
  Demux2/2 -> Thruster Analogue Force Calculator/5(Ty)
  T_d/1 -> Demux2/1  "T_d"
  F_d/1 -> Demux1/1  "F_d"
  Thruster Analogue Force Calculator/2(t_open) -> Thruster PWM Force Calculator/3(t_open)  "t_open"
  Thruster Analogue Force Calculator/1(Ft) -> Thruster PWM Force Calculator/2(Ft)  "F_thruster"
  Clock/1 -> Thruster PWM Force Calculator/1(time)
  Thruster PWM Force Calculator/1(Ftp) -> To Workspace/1  "F_thruster_pwm"
  Thruster Analogue Force Calculator/3(Forces) -> Demux3/1  "F"
  Demux3/1 -> Mux/1
  Demux3/2 -> Mux/2
  Demux3/3 -> Mux/3
  Demux3/4 -> Mux1/1
  Demux3/5 -> Mux1/2
  Demux3/6 -> Mux1/3
  Mux/1 -> F/1  "F"
  Mux1/1 -> T/1  "T"

== system Simulink_Model/V Matrix Calculation ==
  ω_rw : Inport
  ω : Inport  Port=2
  I_rw_z : Gain  Gain=I_rw_z
  I_sys : Gain  Gain=I_sys  Multiplication=Matrix(K*u) (u vector)
  R_1_to_0 : Gain  Gain=R_1_to_0  Multiplication=Matrix(K*u) (u vector)
  Sum : Sum  Inputs=++|
  ω x (I*ω) : vrlib/Utilities/Cross Product
      settings: SourceProductBaseCode=VR
  ω x h : vrlib/Utilities/Cross Product
      settings: SourceProductBaseCode=VR
  V : Outport
  wires:
  ω x (I*ω)/1 -> Sum/1  "ω x (I*ω)"
  ω x h/1 -> Sum/2  "ω x h"
  Sum/1 -> V/1  "V Matrix"
  ω/1 -> ω x h/1, I_sys/1, ω x (I*ω)/1  "ω"
  I_sys/1 -> ω x (I*ω)/2  "I*ω"
  ω_rw/1 -> I_rw_z/1
  I_rw_z/1 -> R_1_to_0/1
  R_1_to_0/1 -> ω x h/2

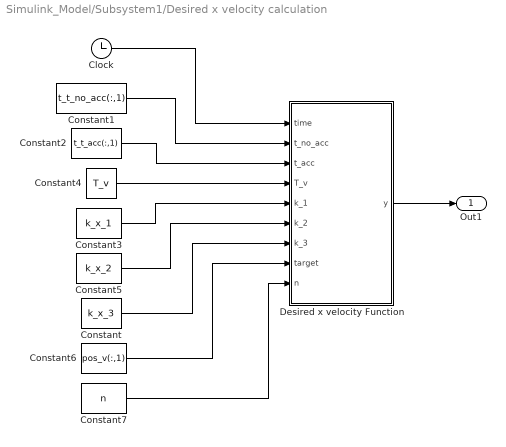
== system Simulink_Model/Subsystem1/Desired x velocity calculation ==
  Clock : Clock
  Constant : Constant  Value=k_x_3
  Constant1 : Constant  Value=t_t_no_acc(:,1)
  Constant2 : Constant  Value=t_t_acc(:,1)
  Constant3 : Constant  Value=k_x_1
  Constant4 : Constant  Value=T_v
  Constant5 : Constant  Value=k_x_2
  Constant6 : Constant  Value=pos_v(:,1)
  Constant7 : Constant  Value=n
  Desired x velocity Function : MATLAB Function  TreatAsAtomicUnit=on
  Out1 : Outport
  wires:
  Clock/1 -> Desired x velocity Function/1(time)
  Desired x velocity Function/1(y) -> Out1/1
  Constant1/1 -> Desired x velocity Function/2(t_no_acc)
  Constant2/1 -> Desired x velocity Function/3(t_acc)
  Constant4/1 -> Desired x velocity Function/4(T_v)
  Constant/1 -> Desired x velocity Function/7(k_3)
  Constant5/1 -> Desired x velocity Function/6(k_2)
  Constant3/1 -> Desired x velocity Function/5(k_1)
  Constant6/1 -> Desired x velocity Function/8(target)
  Constant7/1 -> Desired x velocity Function/9(n)

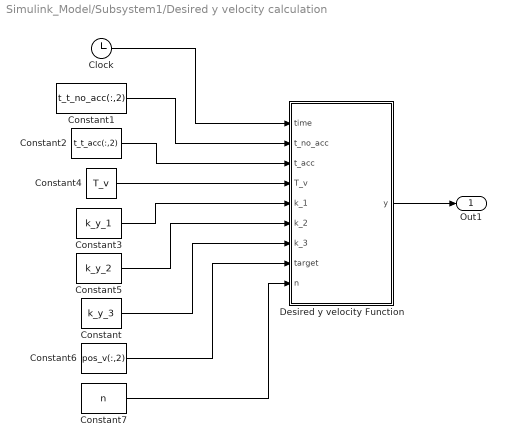
== system Simulink_Model/Subsystem1/Desired y velocity calculation ==
  Clock : Clock
  Constant : Constant  Value=k_y_3
  Constant1 : Constant  Value=t_t_no_acc(:,2)
  Constant2 : Constant  Value=t_t_acc(:,2)
  Constant3 : Constant  Value=k_y_1
  Constant4 : Constant  Value=T_v
  Constant5 : Constant  Value=k_y_2
  Constant6 : Constant  Value=pos_v(:,2)
  Constant7 : Constant  Value=n
  Desired y velocity Function : MATLAB Function  TreatAsAtomicUnit=on
  Out1 : Outport
  wires:
  Constant5/1 -> Desired y velocity Function/6(k_2)
  Constant4/1 -> Desired y velocity Function/4(T_v)
  Constant1/1 -> Desired y velocity Function/2(t_no_acc)
  Desired y velocity Function/1(y) -> Out1/1
  Constant6/1 -> Desired y velocity Function/8(target)
  Constant3/1 -> Desired y velocity Function/5(k_1)
  Clock/1 -> Desired y velocity Function/1(time)
  Constant2/1 -> Desired y velocity Function/3(t_acc)
  Constant/1 -> Desired y velocity Function/7(k_3)
  Constant7/1 -> Desired y velocity Function/9(n)

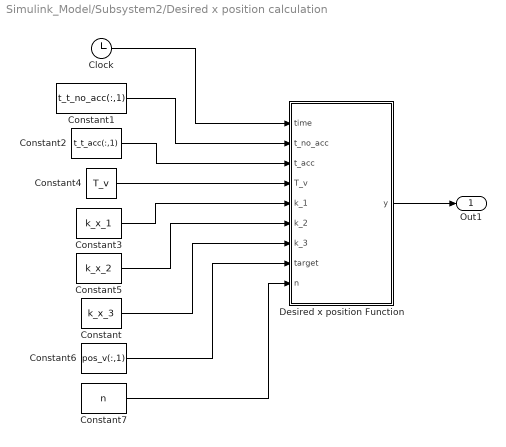
== system Simulink_Model/Subsystem2/Desired x position calculation ==
  Clock : Clock
  Constant : Constant  Value=k_x_3
  Constant1 : Constant  Value=t_t_no_acc(:,1)
  Constant2 : Constant  Value=t_t_acc(:,1)
  Constant3 : Constant  Value=k_x_1
  Constant4 : Constant  Value=T_v
  Constant5 : Constant  Value=k_x_2
  Constant6 : Constant  Value=pos_v(:,1)
  Constant7 : Constant  Value=n
  Desired x position Function : MATLAB Function  TreatAsAtomicUnit=on
  Out1 : Outport
  wires:
  Clock/1 -> Desired x position Function/1(time)
  Desired x position Function/1(y) -> Out1/1
  Constant1/1 -> Desired x position Function/2(t_no_acc)
  Constant2/1 -> Desired x position Function/3(t_acc)
  Constant4/1 -> Desired x position Function/4(T_v)
  Constant/1 -> Desired x position Function/7(k_3)
  Constant5/1 -> Desired x position Function/6(k_2)
  Constant3/1 -> Desired x position Function/5(k_1)
  Constant6/1 -> Desired x position Function/8(target)
  Constant7/1 -> Desired x position Function/9(n)

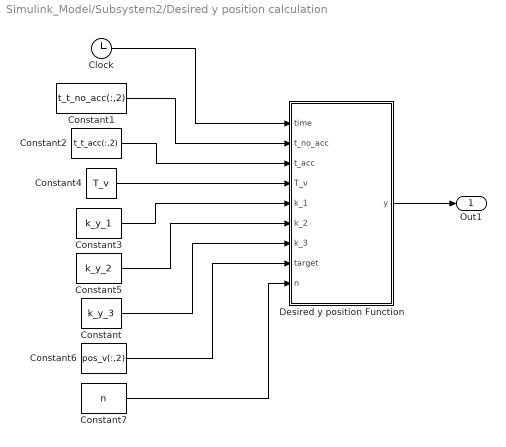
== system Simulink_Model/Subsystem2/Desired y position calculation ==
  Clock : Clock
  Constant : Constant  Value=k_y_3
  Constant1 : Constant  Value=t_t_no_acc(:,2)
  Constant2 : Constant  Value=t_t_acc(:,2)
  Constant3 : Constant  Value=k_y_1
  Constant4 : Constant  Value=T_v
  Constant5 : Constant  Value=k_y_2
  Constant6 : Constant  Value=pos_v(:,2)
  Constant7 : Constant  Value=n
  Desired y position Function : MATLAB Function  TreatAsAtomicUnit=on
  Out1 : Outport
  wires:
  Constant5/1 -> Desired y position Function/6(k_2)
  Constant4/1 -> Desired y position Function/4(T_v)
  Constant1/1 -> Desired y position Function/2(t_no_acc)
  Desired y position Function/1(y) -> Out1/1
  Constant6/1 -> Desired y position Function/8(target)
  Constant3/1 -> Desired y position Function/5(k_1)
  Clock/1 -> Desired y position Function/1(time)
  Constant2/1 -> Desired y position Function/3(t_acc)
  Constant/1 -> Desired y position Function/7(k_3)
  Constant7/1 -> Desired y position Function/9(n)

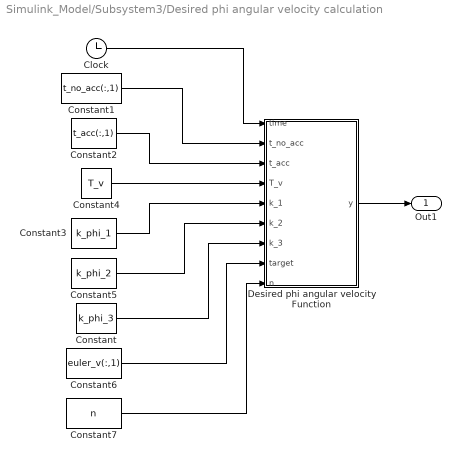
== system Simulink_Model/Subsystem3/Desired phi angular velocity calculation ==
  Clock : Clock
  Constant : Constant  Value=k_phi_3
  Constant1 : Constant  Value=t_no_acc(:,1)
  Constant2 : Constant  Value=t_acc(:,1)
  Constant3 : Constant  Value=k_phi_1
  Constant4 : Constant  Value=T_v
  Constant5 : Constant  Value=k_phi_2
  Constant6 : Constant  Value=euler_v(:,1)
  Constant7 : Constant  Value=n
  Desired phi angular velocity Function : MATLAB Function  TreatAsAtomicUnit=on
  Out1 : Outport
  wires:
  Clock/1 -> Desired phi angular velocity Function/1(time)
  Desired phi angular velocity Function/1(y) -> Out1/1
  Constant1/1 -> Desired phi angular velocity Function/2(t_no_acc)
  Constant2/1 -> Desired phi angular velocity Function/3(t_acc)
  Constant4/1 -> Desired phi angular velocity Function/4(T_v)
  Constant/1 -> Desired phi angular velocity Function/7(k_3)
  Constant5/1 -> Desired phi angular velocity Function/6(k_2)
  Constant3/1 -> Desired phi angular velocity Function/5(k_1)
  Constant6/1 -> Desired phi angular velocity Function/8(target)
  Constant7/1 -> Desired phi angular velocity Function/9(n)

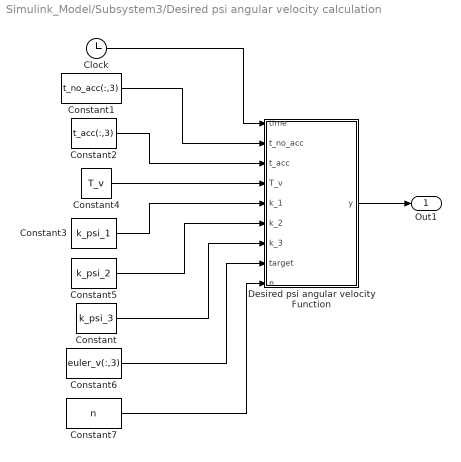
== system Simulink_Model/Subsystem3/Desired psi angular velocity calculation ==
  Clock : Clock
  Constant : Constant  Value=k_psi_3
  Constant1 : Constant  Value=t_no_acc(:,3)
  Constant2 : Constant  Value=t_acc(:,3)
  Constant3 : Constant  Value=k_psi_1
  Constant4 : Constant  Value=T_v
  Constant5 : Constant  Value=k_psi_2
  Constant6 : Constant  Value=euler_v(:,3)
  Constant7 : Constant  Value=n
  Desired psi angular velocity Function : MATLAB Function  TreatAsAtomicUnit=on
  Out1 : Outport
  wires:
  Constant1/1 -> Desired psi angular velocity Function/2(t_no_acc)
  Constant5/1 -> Desired psi angular velocity Function/6(k_2)
  Constant3/1 -> Desired psi angular velocity Function/5(k_1)
  Constant2/1 -> Desired psi angular velocity Function/3(t_acc)
  Desired psi angular velocity Function/1(y) -> Out1/1
  Constant4/1 -> Desired psi angular velocity Function/4(T_v)
  Constant/1 -> Desired psi angular velocity Function/7(k_3)
  Clock/1 -> Desired psi angular velocity Function/1(time)
  Constant7/1 -> Desired psi angular velocity Function/9(n)
  Constant6/1 -> Desired psi angular velocity Function/8(target)

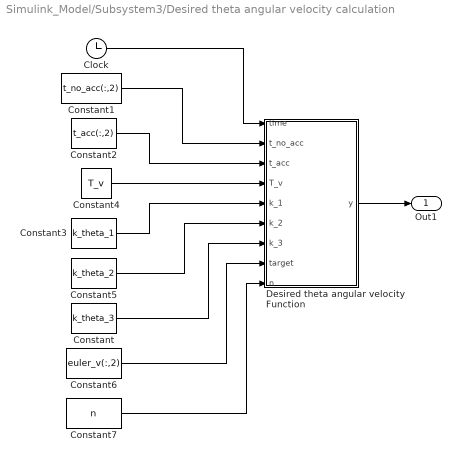
== system Simulink_Model/Subsystem3/Desired theta angular velocity calculation ==
  Clock : Clock
  Constant : Constant  Value=k_theta_3
  Constant1 : Constant  Value=t_no_acc(:,2)
  Constant2 : Constant  Value=t_acc(:,2)
  Constant3 : Constant  Value=k_theta_1
  Constant4 : Constant  Value=T_v
  Constant5 : Constant  Value=k_theta_2
  Constant6 : Constant  Value=euler_v(:,2)
  Constant7 : Constant  Value=n
  Desired theta angular velocity Function : MATLAB Function  TreatAsAtomicUnit=on
  Out1 : Outport
  wires:
  Constant1/1 -> Desired theta angular velocity Function/2(t_no_acc)
  Constant5/1 -> Desired theta angular velocity Function/6(k_2)
  Constant3/1 -> Desired theta angular velocity Function/5(k_1)
  Constant2/1 -> Desired theta angular velocity Function/3(t_acc)
  Desired theta angular velocity Function/1(y) -> Out1/1
  Constant4/1 -> Desired theta angular velocity Function/4(T_v)
  Constant/1 -> Desired theta angular velocity Function/7(k_3)
  Clock/1 -> Desired theta angular velocity Function/1(time)
  Constant7/1 -> Desired theta angular velocity Function/9(n)
  Constant6/1 -> Desired theta angular velocity Function/8(target)

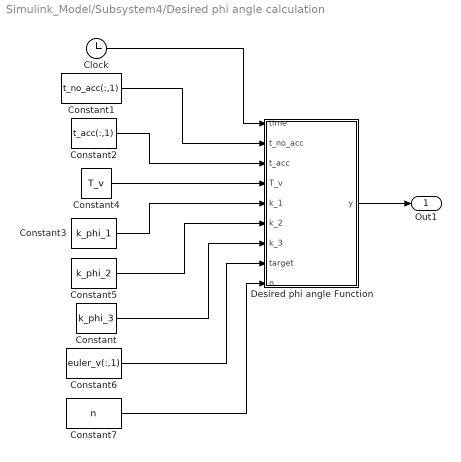
== system Simulink_Model/Subsystem4/Desired phi angle calculation ==
  Clock : Clock
  Constant : Constant  Value=k_phi_3
  Constant1 : Constant  Value=t_no_acc(:,1)
  Constant2 : Constant  Value=t_acc(:,1)
  Constant3 : Constant  Value=k_phi_1
  Constant4 : Constant  Value=T_v
  Constant5 : Constant  Value=k_phi_2
  Constant6 : Constant  Value=euler_v(:,1)
  Constant7 : Constant  Value=n
  Desired phi angle Function : MATLAB Function  TreatAsAtomicUnit=on
  Out1 : Outport
  wires:
  Clock/1 -> Desired phi angle Function/1(time)
  Desired phi angle Function/1(y) -> Out1/1
  Constant1/1 -> Desired phi angle Function/2(t_no_acc)
  Constant2/1 -> Desired phi angle Function/3(t_acc)
  Constant4/1 -> Desired phi angle Function/4(T_v)
  Constant/1 -> Desired phi angle Function/7(k_3)
  Constant5/1 -> Desired phi angle Function/6(k_2)
  Constant3/1 -> Desired phi angle Function/5(k_1)
  Constant6/1 -> Desired phi angle Function/8(target)
  Constant7/1 -> Desired phi angle Function/9(n)
